simulink model "Ieee14_CC"  (R2023b)
settings: Solver=ode1  StartTime=0.0  StopTime=600  FixedStep=1e-3  MaxStep=1e-4  RelTol=1e-3
model workspace (MAT data in the model file):
  pruebaValor = 0
undefined symbols (not defined in the file or in its folder): f
libraries: spsThreePhaseVIMeasurementLib x39, spsThreePhaseBreakerLib x21, spsLoadFlowBusLib x19, spsThreePhaseSeriesRLCBranchLib x16, spsThreePhaseFaultLib x16, source_mod x14, instrumentlib x8, spsThreePhaseTransformerTwoWindingsLib x4, spsThreePhaseSourceLib x2, sps_lib x1
(part 2 of 2)

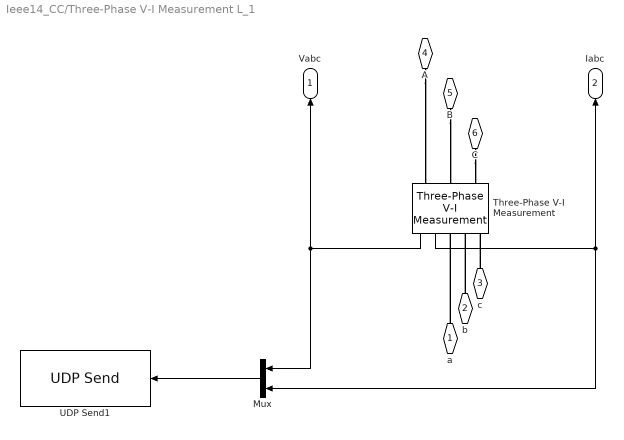
== system Ieee14_CC/Three-Phase V-I Measurement L_1 ==
  Mux : Mux  Inputs=2
  Three-Phase V-I Measurement : spsThreePhaseVIMeasurementLib/Three-Phase V-I Measurement  VoltageMeasurement=phase-to-ground  SetLabelV=off  LabelV=Vabc  Vpu=on  VpuLL=off  CurrentMeasurement=yes  SetLabelI=off  LabelI=Iabc  Ipu=on  Pbase=100e6  Vbase=69e3  OutputType=Complex  PhasorSimulation=off  PSBequivalent=0
  UDP Send1 : instrumentlib/UDP Send  Host=10.0.0.1  Port=10001  LocalAddress=0.0.0.0  LocalPort=-1  EnablePortSharing=off  OutputDatagramPacketSize=512  ByteOrder=big-endian  EnableBlockingMode=on  SimulateUsing=Interpreted execution
  a : PMIOPort  Side=Left
  b : PMIOPort  Port=2  Side=Left
  c : PMIOPort  Port=3  Side=Left
  A : PMIOPort  Port=4  Side=Right
  B : PMIOPort  Port=5  Side=Right
  C : PMIOPort  Port=6  Side=Right
  Vabc : Outport
  Iabc : Outport  Port=2
  wires:
  Three-Phase V-I Measurement/1 -> Vabc/1, Mux/1
  Three-Phase V-I Measurement/2 -> Mux/2, Iabc/1
  Mux/1 -> UDP Send1/1
  connections:
  b/RConn1 -- Three-Phase V-I Measurement/RConn2
  a/RConn1 -- Three-Phase V-I Measurement/RConn1
  c/RConn1 -- Three-Phase V-I Measurement/RConn3
  A/RConn1 -- Three-Phase V-I Measurement/LConn1
  B/RConn1 -- Three-Phase V-I Measurement/LConn2
  C/RConn1 -- Three-Phase V-I Measurement/LConn3

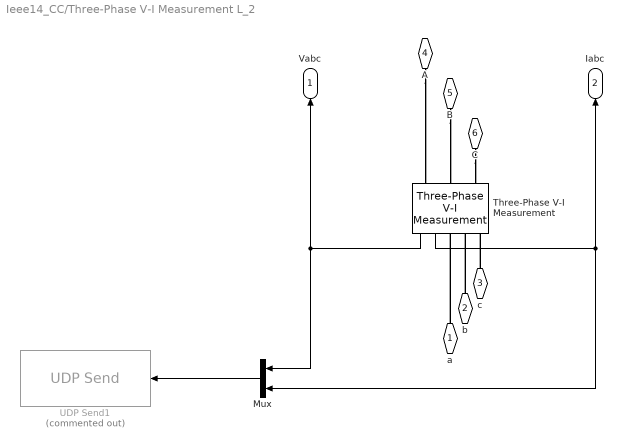
== system Ieee14_CC/Three-Phase V-I Measurement L_2 ==
  Mux : Mux  Inputs=2
  Three-Phase V-I Measurement : spsThreePhaseVIMeasurementLib/Three-Phase V-I Measurement  VoltageMeasurement=phase-to-ground  SetLabelV=off  LabelV=Vabc  Vpu=on  VpuLL=off  CurrentMeasurement=yes  SetLabelI=off  LabelI=Iabc  Ipu=on  Pbase=100e6  Vbase=69e3  OutputType=Complex  PhasorSimulation=off  PSBequivalent=0
  UDP Send1 : instrumentlib/UDP Send  Commented=on  Host=10.0.255.255  Port=10002  LocalAddress=0.0.0.0  LocalPort=-1  EnablePortSharing=off  OutputDatagramPacketSize=512  ByteOrder=big-endian  EnableBlockingMode=on  SimulateUsing=Interpreted execution
  a : PMIOPort  Side=Left
  b : PMIOPort  Port=2  Side=Left
  c : PMIOPort  Port=3  Side=Left
  A : PMIOPort  Port=4  Side=Right
  B : PMIOPort  Port=5  Side=Right
  C : PMIOPort  Port=6  Side=Right
  Vabc : Outport
  Iabc : Outport  Port=2
  wires:
  Three-Phase V-I Measurement/1 -> Vabc/1, Mux/1
  Three-Phase V-I Measurement/2 -> Mux/2, Iabc/1
  Mux/1 -> UDP Send1/1
  connections:
  b/RConn1 -- Three-Phase V-I Measurement/RConn2
  a/RConn1 -- Three-Phase V-I Measurement/RConn1
  c/RConn1 -- Three-Phase V-I Measurement/RConn3
  A/RConn1 -- Three-Phase V-I Measurement/LConn1
  B/RConn1 -- Three-Phase V-I Measurement/LConn2
  C/RConn1 -- Three-Phase V-I Measurement/LConn3

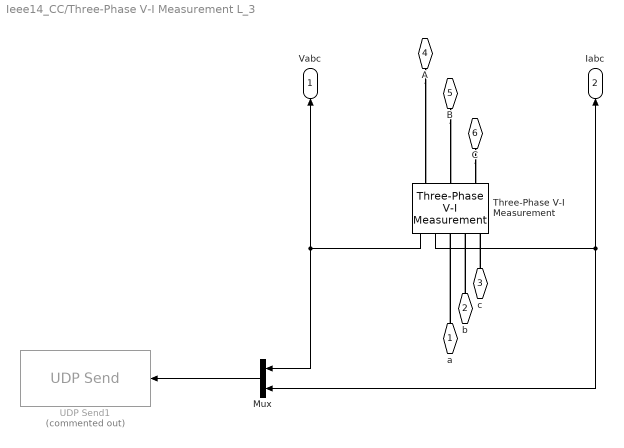
== system Ieee14_CC/Three-Phase V-I Measurement L_3  ==
  Mux : Mux  Inputs=2
  Three-Phase V-I Measurement : spsThreePhaseVIMeasurementLib/Three-Phase V-I Measurement  VoltageMeasurement=phase-to-ground  SetLabelV=off  LabelV=Vabc  Vpu=on  VpuLL=off  CurrentMeasurement=yes  SetLabelI=off  LabelI=Iabc  Ipu=on  Pbase=100e6  Vbase=69e3  OutputType=Complex  PhasorSimulation=off  PSBequivalent=0
  UDP Send1 : instrumentlib/UDP Send  Commented=on  Host=10.0.255.255  Port=10003  LocalAddress=0.0.0.0  LocalPort=-1  EnablePortSharing=off  OutputDatagramPacketSize=512  ByteOrder=big-endian  EnableBlockingMode=on  SimulateUsing=Interpreted execution
  a : PMIOPort  Side=Left
  b : PMIOPort  Port=2  Side=Left
  c : PMIOPort  Port=3  Side=Left
  A : PMIOPort  Port=4  Side=Right
  B : PMIOPort  Port=5  Side=Right
  C : PMIOPort  Port=6  Side=Right
  Vabc : Outport
  Iabc : Outport  Port=2
  wires:
  Three-Phase V-I Measurement/1 -> Vabc/1, Mux/1
  Three-Phase V-I Measurement/2 -> Mux/2, Iabc/1
  Mux/1 -> UDP Send1/1
  connections:
  b/RConn1 -- Three-Phase V-I Measurement/RConn2
  a/RConn1 -- Three-Phase V-I Measurement/RConn1
  c/RConn1 -- Three-Phase V-I Measurement/RConn3
  A/RConn1 -- Three-Phase V-I Measurement/LConn1
  B/RConn1 -- Three-Phase V-I Measurement/LConn2
  C/RConn1 -- Three-Phase V-I Measurement/LConn3

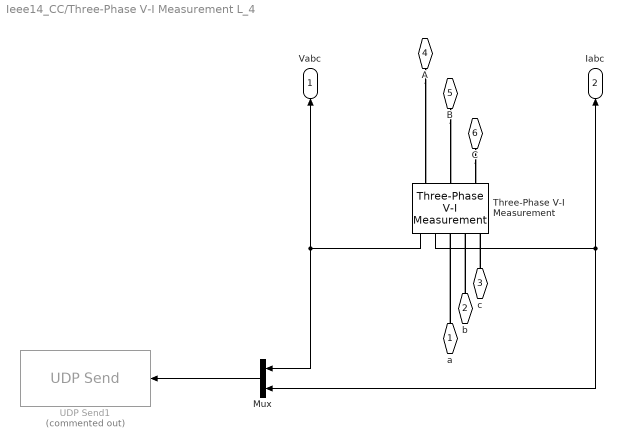
== system Ieee14_CC/Three-Phase V-I Measurement L_4 ==
  Mux : Mux  Inputs=2
  Three-Phase V-I Measurement : spsThreePhaseVIMeasurementLib/Three-Phase V-I Measurement  VoltageMeasurement=phase-to-ground  SetLabelV=off  LabelV=Vabc  Vpu=on  VpuLL=off  CurrentMeasurement=yes  SetLabelI=off  LabelI=Iabc  Ipu=on  Pbase=100e6  Vbase=69e3  OutputType=Complex  PhasorSimulation=off  PSBequivalent=0
  UDP Send1 : instrumentlib/UDP Send  Commented=on  Host=10.0.255.255  Port=10004  LocalAddress=0.0.0.0  LocalPort=-1  EnablePortSharing=off  OutputDatagramPacketSize=512  ByteOrder=big-endian  EnableBlockingMode=on  SimulateUsing=Interpreted execution
  a : PMIOPort  Side=Left
  b : PMIOPort  Port=2  Side=Left
  c : PMIOPort  Port=3  Side=Left
  A : PMIOPort  Port=4  Side=Right
  B : PMIOPort  Port=5  Side=Right
  C : PMIOPort  Port=6  Side=Right
  Vabc : Outport
  Iabc : Outport  Port=2
  wires:
  Three-Phase V-I Measurement/1 -> Vabc/1, Mux/1
  Three-Phase V-I Measurement/2 -> Mux/2, Iabc/1
  Mux/1 -> UDP Send1/1
  connections:
  b/RConn1 -- Three-Phase V-I Measurement/RConn2
  a/RConn1 -- Three-Phase V-I Measurement/RConn1
  c/RConn1 -- Three-Phase V-I Measurement/RConn3
  A/RConn1 -- Three-Phase V-I Measurement/LConn1
  B/RConn1 -- Three-Phase V-I Measurement/LConn2
  C/RConn1 -- Three-Phase V-I Measurement/LConn3

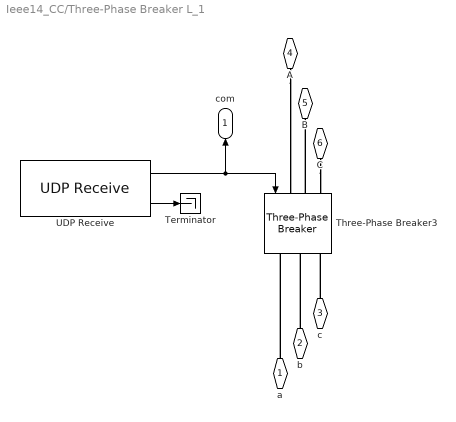
== system Ieee14_CC/Three-Phase Breaker L_1 ==
  Terminator : Terminator
  Three-Phase Breaker3 : spsThreePhaseBreakerLib/Three-Phase Breaker  InitialState=closed  SwitchA=on  SwitchB=on  SwitchC=on  SwitchTimes=[0.2]  External=on  BreakerResistance=0.01  SnubberResistance=1e6  SnubberCapacitance=inf  Measurements=Breaker voltages and currents
  UDP Receive : instrumentlib/UDP Receive  LocalAddress=0.0.0.0  LocalPort=30001  EnablePortSharing=off  Host=10.0.1.2  Port=30001  GetLatestData=off  DataSize=[ 1, 1 ]  DataType=uint16  ASCIIFormatting=%f,  Terminator=LF  CustomTerminator=10  ByteOrder=big-endian  EnableBlockingMode=off  Timeout=10  SampleTime=0.01  SimulateUsing=Interpreted execution
  a : PMIOPort  Side=Left
  b : PMIOPort  Port=2  Side=Left
  c : PMIOPort  Port=3  Side=Left
  A : PMIOPort  Port=4  Side=Right
  B : PMIOPort  Port=5  Side=Right
  C : PMIOPort  Port=6  Side=Right
  com : Outport
  wires:
  UDP Receive/1 -> com/1, Three-Phase Breaker3/1
  UDP Receive/2 -> Terminator/1
  connections:
  b/RConn1 -- Three-Phase Breaker3/RConn2
  c/RConn1 -- Three-Phase Breaker3/RConn3
  A/RConn1 -- Three-Phase Breaker3/LConn1
  Three-Phase Breaker3/LConn2 -- B/RConn1
  C/RConn1 -- Three-Phase Breaker3/LConn3
  a/RConn1 -- Three-Phase Breaker3/RConn1

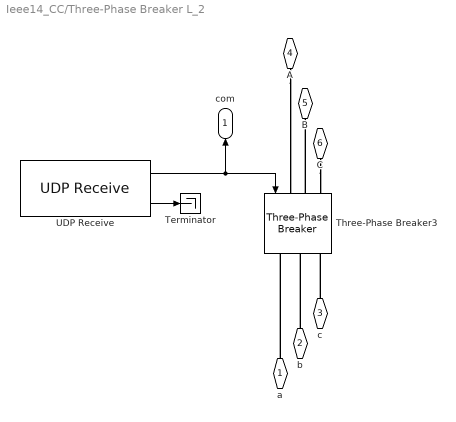
== system Ieee14_CC/Three-Phase Breaker L_2 ==
  Terminator : Terminator
  Three-Phase Breaker3 : spsThreePhaseBreakerLib/Three-Phase Breaker  InitialState=closed  SwitchA=on  SwitchB=on  SwitchC=on  SwitchTimes=[0.2]  External=on  BreakerResistance=0.01  SnubberResistance=1e6  SnubberCapacitance=inf  Measurements=Breaker voltages and currents
  UDP Receive : instrumentlib/UDP Receive  LocalAddress=0.0.0.0  LocalPort=30002  EnablePortSharing=off  Host=10.0.2.2  Port=30002  GetLatestData=off  DataSize=[ 1, 1 ]  DataType=uint16  ASCIIFormatting=%f,  Terminator=LF  CustomTerminator=10  ByteOrder=big-endian  EnableBlockingMode=off  Timeout=10  SampleTime=0.01  SimulateUsing=Interpreted execution
  a : PMIOPort  Side=Left
  b : PMIOPort  Port=2  Side=Left
  c : PMIOPort  Port=3  Side=Left
  A : PMIOPort  Port=4  Side=Right
  B : PMIOPort  Port=5  Side=Right
  C : PMIOPort  Port=6  Side=Right
  com : Outport
  wires:
  UDP Receive/1 -> com/1, Three-Phase Breaker3/1
  UDP Receive/2 -> Terminator/1
  connections:
  b/RConn1 -- Three-Phase Breaker3/RConn2
  c/RConn1 -- Three-Phase Breaker3/RConn3
  A/RConn1 -- Three-Phase Breaker3/LConn1
  Three-Phase Breaker3/LConn2 -- B/RConn1
  C/RConn1 -- Three-Phase Breaker3/LConn3
  a/RConn1 -- Three-Phase Breaker3/RConn1

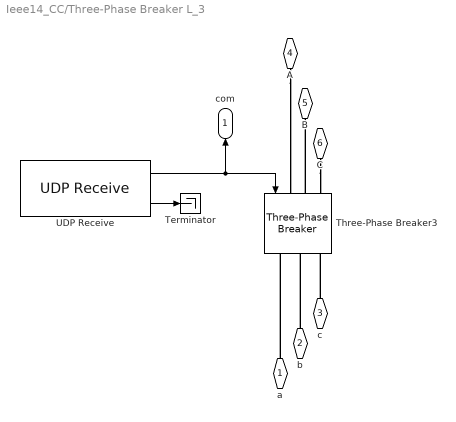
== system Ieee14_CC/Three-Phase Breaker L_3 ==
  Terminator : Terminator
  Three-Phase Breaker3 : spsThreePhaseBreakerLib/Three-Phase Breaker  InitialState=closed  SwitchA=on  SwitchB=on  SwitchC=on  SwitchTimes=[0.2]  External=on  BreakerResistance=0.01  SnubberResistance=1e6  SnubberCapacitance=inf  Measurements=Breaker voltages and currents
  UDP Receive : instrumentlib/UDP Receive  LocalAddress=0.0.0.0  LocalPort=30003  EnablePortSharing=off  Host=10.0.3.2  Port=30003  GetLatestData=off  DataSize=[ 1, 1 ]  DataType=uint16  ASCIIFormatting=%f,  Terminator=LF  CustomTerminator=10  ByteOrder=big-endian  EnableBlockingMode=off  Timeout=10  SampleTime=0.01  SimulateUsing=Interpreted execution
  a : PMIOPort  Side=Left
  b : PMIOPort  Port=2  Side=Left
  c : PMIOPort  Port=3  Side=Left
  A : PMIOPort  Port=4  Side=Right
  B : PMIOPort  Port=5  Side=Right
  C : PMIOPort  Port=6  Side=Right
  com : Outport
  wires:
  UDP Receive/1 -> com/1, Three-Phase Breaker3/1
  UDP Receive/2 -> Terminator/1
  connections:
  b/RConn1 -- Three-Phase Breaker3/RConn2
  c/RConn1 -- Three-Phase Breaker3/RConn3
  A/RConn1 -- Three-Phase Breaker3/LConn1
  Three-Phase Breaker3/LConn2 -- B/RConn1
  C/RConn1 -- Three-Phase Breaker3/LConn3
  a/RConn1 -- Three-Phase Breaker3/RConn1

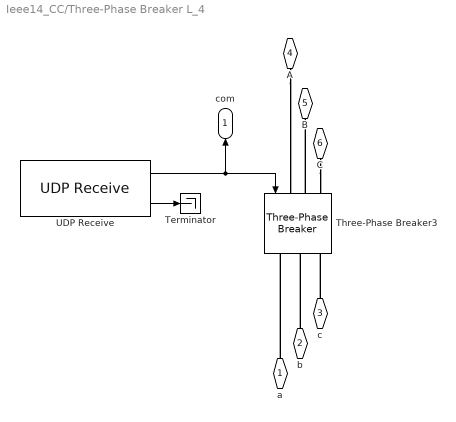
== system Ieee14_CC/Three-Phase Breaker L_4 ==
  Terminator : Terminator
  Three-Phase Breaker3 : spsThreePhaseBreakerLib/Three-Phase Breaker  InitialState=closed  SwitchA=on  SwitchB=on  SwitchC=on  SwitchTimes=[0.2]  External=on  BreakerResistance=0.01  SnubberResistance=1e6  SnubberCapacitance=inf  Measurements=Breaker voltages and currents
  UDP Receive : instrumentlib/UDP Receive  LocalAddress=0.0.0.0  LocalPort=30004  EnablePortSharing=off  Host=10.0.4.2  Port=30004  GetLatestData=off  DataSize=[ 1, 1 ]  DataType=uint16  ASCIIFormatting=%f,  Terminator=LF  CustomTerminator=10  ByteOrder=big-endian  EnableBlockingMode=off  Timeout=10  SampleTime=0.01  SimulateUsing=Interpreted execution
  a : PMIOPort  Side=Left
  b : PMIOPort  Port=2  Side=Left
  c : PMIOPort  Port=3  Side=Left
  A : PMIOPort  Port=4  Side=Right
  B : PMIOPort  Port=5  Side=Right
  C : PMIOPort  Port=6  Side=Right
  com : Outport
  wires:
  UDP Receive/1 -> com/1, Three-Phase Breaker3/1
  UDP Receive/2 -> Terminator/1
  connections:
  b/RConn1 -- Three-Phase Breaker3/RConn2
  c/RConn1 -- Three-Phase Breaker3/RConn3
  A/RConn1 -- Three-Phase Breaker3/LConn1
  Three-Phase Breaker3/LConn2 -- B/RConn1
  C/RConn1 -- Three-Phase Breaker3/LConn3
  a/RConn1 -- Three-Phase Breaker3/RConn1

== matlab function Ieee14_CC/InicioFcn ==
  settings: sampleTime=0
  data: u input
function fcn(u)

%{

Funcion: inicioFcn

Detalles: Funcion de inicializacion de la red. Se ejecuta 1 sola vez. 
Llama a la funcion resetRed externa que inicializa los valores de la red.

Adicional: Para evitar cualquier mensaje de warning, se anulan desde la
linea warning('off','all'). A pesar del warning, no es un problema para el
funcionamiento de la red

%}

% - - - - - - - - - - - - - - - - - - - - - - - - -

% Coder
coder.extrinsic('resetRed');
coder.extrinsic('warning');

% - - - - - - - - - - - - - - - - - - - - - - - - -

% Resetar
if u == 0
    resetRed();
    warning('off','all');
end

% - - - - - - - - - - - - - - - - - - - - - - - - -
end

== matlab function Ieee14_CC/CC ==
  settings: updateMethod=DISCRETE  sampleTime=10
function fcn()

    %{
    
    Funcion CC: cortocircuitos. 
    
    Detalles: Esta funcion se encarga de ocasionar las cortocircuitos a lo
    largo de la simulacion.
    
    Importante: En edit Data, se debe ajustar cada x tiempo que se quiera
    entrar en esta funcion. Si el valor es 5 segundos, su compartimiento es: 
    
    T = 5s --> Se activa CC
    T = 10s --> Se desactiva CC
    T = 15s --> Se activa CC
    T = 20s --> Se desactiva CC
    ... ... ...
    
    %}
    
    % - - - - - - - - - - - - - - - - - - - - - - - - -
    
    % coders
    coder.extrinsic('mat2str');
    coder.extrinsic('set_param');
    
    % - - - - - - - - - - - - - - - - - - - - - - - - -
    
    % Ajustes de variables
    % Si saltar es 1, no se activaran CC. Poner a 0. 
    saltar = 0;
    
    % - - - - - - - - - - - - - - - - - - - - - - - - -
    
    % = = = = = = = = = = = = = = = = = = = = = = = = =
    % = = = = = = = = = = = = = = = = = = = = = = = = =
    % - - - - - - - - Codigo - - - - - - - - - - - - - 
    % = = = = = = = = = = = = = = = = = = = = = = = = =
    % = = = = = = = = = = = = = = = = = = = = = = = = =
    
    % - - - - - - - - - - - - - - - - - - - - - - - - -
    
    % Activar o desactivar funcion
    if saltar == 1
        return
    end
    
    % - - - - - - - - - - - - - - - - - - - - - - - - -
    
    % Variables persistents
    
    % ataque: si es 1 se produce el cortocircuito (cc)
    persistent ataque
    if isempty(ataque)
       ataque = 0;
       return
    end
    
    % lineaCC: linea que tiene cortocircuito
    persistent lineaCC;
    if isempty(lineaCC)
        lineaCC = 0;
    end
    
    % - - - - - - - - - - - - - - - - - - - - - - - - -
    
    % direccion del modelo
    direccion = "Ieee14_CC/";
    
    % - - - - - - - - - - - - - - - - - - - - - - - - -
    
    % Restaurar ataque
    if ataque == 1
        if lineaCC == 1
            linea = "B1_L5";
            aux = direccion + "CC_" + linea;
            set_param(aux, 'Value', mat2str(0));
        end
        if lineaCC == 2
            linea = "B1_L4";
            aux = direccion + "CC_" + linea;
            set_param(aux, 'Value', mat2str(0));
        end
        if lineaCC == 3
            linea = "B2_G1";
            aux = direccion + "CC_" + linea;
            set_param(aux, 'Value', mat2str(0));
        end
        if lineaCC == 4
            linea = "B2_L5";
            aux = direccion + "CC_" + linea;
            set_param(aux, 'Value', mat2str(0));
        end
        if lineaCC == 5
            linea = "B2_L4";
            aux = direccion + "CC_" + linea;
            set_param(aux, 'Value', mat2str(0));
        end
        if lineaCC == 6
            linea = "B2_G3";
            aux = direccion + "CC_" + linea;
            set_param(aux, 'Value', mat2str(0));
        end
        if lineaCC == 7
            linea = "B3_L4";
            aux = direccion + "CC_" + linea;
            set_param(aux, 'Value', mat2str(0));
        end
        if lineaCC == 8
            linea = "L1";
            aux = direccion + "CC_" + linea;
            set_param(aux, 'Value', mat2str(0));
        end
        if lineaCC == 9
            linea = "L2";
            aux = direccion + "CC_" + linea;
            set_param(aux, 'Value', mat2str(0));
        end
        if lineaCC == 10
            linea = "L3";
            aux = direccion + "CC_" + linea;
            set_param(aux, 'Value', mat2str(0));
        end
        if lineaCC == 11
            linea = "L4";
            aux = direccion + "CC_" + linea;
            set_param(aux, 'Value', mat2str(0));
        end
        if lineaCC == 12
            linea = "B6_L10";
            aux = direccion + "CC_" + linea;
            set_param(aux, 'Value', mat2str(0));
        end
        if lineaCC == 13
            linea = "B6_L14";
            aux = direccion + "CC_" + linea;
            set_param(aux, 'Value', mat2str(0));
        end
        if lineaCC == 14
            linea = "B8_L5";
            aux = direccion + "CC_" + linea;
            set_param(aux, 'Value', mat2str(0));
        end
        if lineaCC == 15
            linea = "B8_L14";
            aux = direccion + "CC_" + linea;
            set_param(aux, 'Value', mat2str(0));
        end
        if lineaCC == 16
            linea = "B8_L10";
            aux = direccion + "CC_" + linea;
            set_param(aux, 'Value', mat2str(0));
        end
    
        ataque = 0;
        disp('=============')
        disp('desconexion CC');
        disp('=============');
        return
    end
    
    % Activar cortocircuito
    
    if ataque == 0
        % linea CC puede ser usado como mucho con 4 lineas al azar. 
        lineaCC = randi(160);
        %lineaCC = 1;
        disp('=======================');
        disp('=======================');
        disp('LineaCC');
        disp(lineaCC);
        disp('=======================');
        disp('=======================');
        if lineaCC == 1
            linea = "B1_L5";
            aux = direccion + "CC_" + linea;
            set_param(aux, 'Value', mat2str(1));
        end
        if lineaCC == 2
            linea = "B1_L4";
            aux = direccion + "CC_" + linea;
            set_param(aux, 'Value', mat2str(1));
        end
        if lineaCC == 3
            linea = "B2_G1";
            aux = direccion + "CC_" + linea;
            set_param(aux, 'Value', mat2str(1));
        end
        if lineaCC == 4
            linea = "B2_L5";
            aux = direccion + "CC_" + linea;
            set_param(aux, 'Value', mat2str(1));
        end
        if lineaCC == 5
            linea = "B2_L4";
            aux = direccion + "CC_" + linea;
            set_param(aux, 'Value', mat2str(1));
        end
        if lineaCC == 6
            linea = "B2_G3";
            aux = direccion + "CC_" + linea;
            set_param(aux, 'Value', mat2str(1));
        end
        if lineaCC == 7
            linea = "B3_L4";
            aux = direccion + "CC_" + linea;
            set_param(aux, 'Value', mat2str(1));
        end
        if lineaCC == 8
            linea = "B6_L11";
            aux = direccion + "CC_" + linea;
            set_param(aux, 'Value', mat2str(1));
        end
        if lineaCC == 9
            linea = "B6_L12";
            aux = direccion + "CC_" + linea;
            set_param(aux, 'Value', mat2str(1));
        end
        if lineaCC == 10
            linea = "B6_L13";
            aux = direccion + "CC_" + linea;
            set_param(aux, 'Value', mat2str(1));
        end
        if lineaCC == 11
            linea = "B6_L13_2";
            aux = direccion + "CC_" + linea;
            set_param(aux, 'Value', mat2str(1));
        end
        if lineaCC == 12
            linea = "B6_L10";
            aux = direccion + "CC_" + linea;
            set_param(aux, 'Value', mat2str(1));
        end
        if lineaCC == 13
            linea = "B6_L14";
            aux = direccion + "CC_" + linea;
            set_param(aux, 'Value', mat2str(1));
        end
        if lineaCC == 14
            linea = "B8_L5";
            aux = direccion + "CC_" + linea;
            set_param(aux, 'Value', mat2str(1));
        end
        if lineaCC == 15
            linea = "B8_L14";
            aux = direccion + "CC_" + linea;
            set_param(aux, 'Value', mat2str(1));
        end
        if lineaCC == 16
            linea = "B8_L10";
            aux = direccion + "CC_" + linea;
            set_param(aux, 'Value', mat2str(1));
        end
        ataque = 1;
        return
    end

end
